simulink model "simu_hdl_1st"  (R2021b)
settings: Solver=VariableStepAuto  StartTime=0.0  StopTime=5e-4  RelTol=1e-3
libraries: hdlsllib x1
settings Model: Creator=Phecda  LastModifiedBy=Phecda

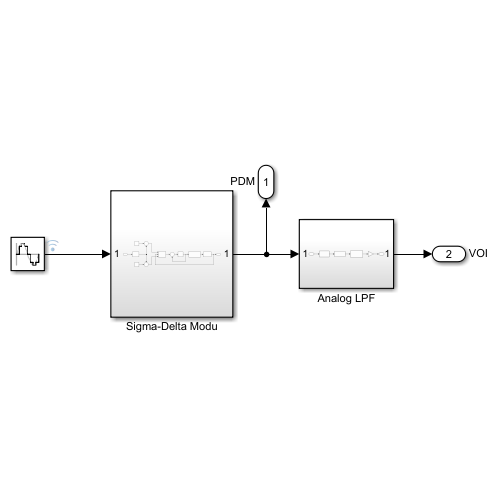
[thumbnail: Simulink's stored preview of the top-level diagram]
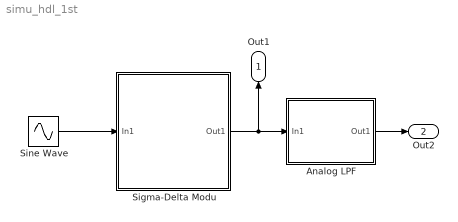
== system simu_hdl_1st ==
  Analog LPF : Subsystem
  Sigma-Delta Modu : Subsystem
  Sine Wave : Sin  Amplitude=30000  Frequency=1e5  SampleTime=0.04e-6
  Out1 : Outport  SignalName=PDM  VectorParamsAs1DForOutWhenUnconnected=off
  Out2 : Outport  Port=2  SignalName=VOI  VectorParamsAs1DForOutWhenUnconnected=off
  wires:
  Sine Wave/1 -> Sigma-Delta Modu/1(In1)
  Sigma-Delta Modu/1(Out1) -> Analog LPF/1(In1), Out1/1
  Analog LPF/1(Out1) -> Out2/1

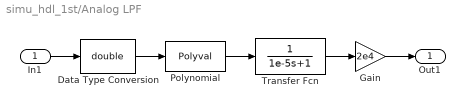
== system simu_hdl_1st/Analog LPF ==
  In1 : Inport
  Data Type Conversion : DataTypeConversion  OutMin=0  OutMax=1  OutDataTypeStr=double  RndMeth=Round
  Gain : Gain  Gain=2e4
  Polynomial : Polyval  Coefs=[2 -1]
  Transfer Fcn : TransferFcn  Denominator=[1e-5 1]
  Out1 : Outport
  wires:
  Gain/1 -> Out1/1
  Transfer Fcn/1 -> Gain/1
  Polynomial/1 -> Transfer Fcn/1
  In1/1 -> Data Type Conversion/1
  Data Type Conversion/1 -> Polynomial/1

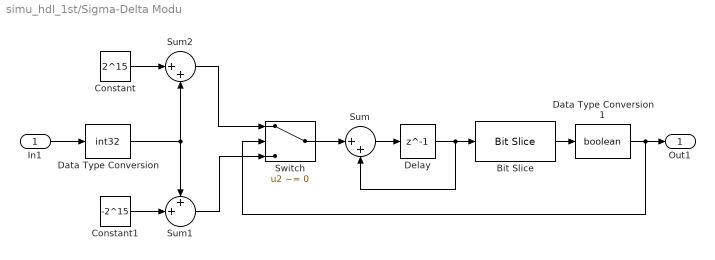
== system simu_hdl_1st/Sigma-Delta Modu ==
  In1 : Inport  SampleTime=0.04e-6
  Bit Slice : hdlsllib/Logic and Bit Operations/Bit Slice  lidx=17  ridx=17
      settings: SourceProductBaseCode=SL
  Constant : Constant  Value=2^15  OutMin=-131071  OutMax=131071  OutDataTypeStr=int32  SampleTime=0.04e-6
  Constant1 : Constant  Value=-2^15  OutMin=-131071  OutMax=131071  OutDataTypeStr=int32  SampleTime=0.04e-6
  Data Type Conversion : DataTypeConversion  OutMin=-131071  OutMax=131071  OutDataTypeStr=int32  RndMeth=Round
  Data Type Conversion1 : DataTypeConversion  OutMin=0  OutMax=1  OutDataTypeStr=boolean  RndMeth=Round
  Delay : Delay  DelayLength=1  InitialCondition=0  SampleTime=0.04e-6
  Sum : Sum  Inputs=|++  AccumDataTypeStr=int32  OutMin=-131071  OutMax=131071  OutDataTypeStr=int32  RndMeth=Round
  Sum1 : Sum  Inputs=++|
  Sum2 : Sum  Inputs=|++
  Switch : Switch  Criteria=u2 ~= 0  OutMin=-131071  OutMax=131071  OutDataTypeStr=int32  RndMeth=Round
  Out1 : Outport  OutMin=0  OutMax=1  SampleTime=0.04e-6
  wires:
  Data Type Conversion1/1 -> Out1/1, Switch/2
  Switch/1 -> Sum/1
  Data Type Conversion/1 -> Sum1/1, Sum2/2
  Constant1/1 -> Sum1/2
  Delay/1 -> Sum/2, Bit Slice/1
  Sum1/1 -> Switch/3
  Sum/1 -> Delay/1
  Constant/1 -> Sum2/1
  Sum2/1 -> Switch/1
  In1/1 -> Data Type Conversion/1
  Bit Slice/1 -> Data Type Conversion1/1
